simulink model "c8t6_antipark_svpwm"  (R2018b)
settings: Solver=FixedStepDiscrete  StartTime=0.0  StopTime=2  FixedStep=0.000001  RelTol=1e-3
libraries: simulink x1
settings Model: Creator=ganlu  LastModifiedBy=ganlu

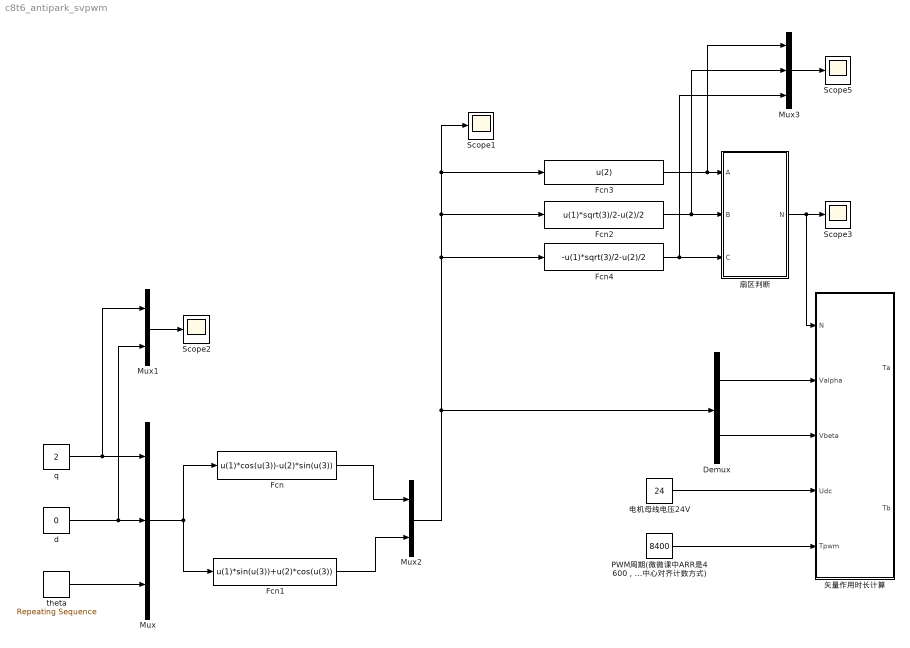
== system c8t6_antipark_svpwm ==
  Demux : Demux  Outputs=2
  Fcn : Fcn  Expr=u(1)*cos(u(3))-u(2)*sin(u(3))
  Fcn1 : Fcn  Expr=u(1)*sin(u(3))+u(2)*cos(u(3))
  Fcn2 : Fcn  Expr=u(1)*sqrt(3)/2-u(2)/2
  Fcn3 : Fcn  Expr=u(2)
  Fcn4 : Fcn  Expr=-u(1)*sqrt(3)/2-u(2)/2
  Mux : Mux  Inputs=3
  Mux1 : Mux  Inputs=2
  Mux2 : Mux  Inputs=2
  Mux3 : Mux  Inputs=3
  "PWM周期(微微课中ARR是4600，中心对齐计数方式) " : Constant  Value=8400
  Scope{1..3,5} (4 alike) : Scope
  d : Constant  Value=0
  q : Constant  Value=2
  theta : simulink/Sources/Repeating Sequence  rep_seq_t=[0 1]  rep_seq_y=[0 2*pi]
  扇区判断 : MATLAB Function  TreatAsAtomicUnit=on
  电机母线电压24V : Constant  Value=24
  矢量作用时长计算 : MATLAB Function  TreatAsAtomicUnit=on
  wires:
  q/1 -> Mux1/1, Mux/1
  d/1 -> Mux1/2, Mux/2
  theta/1 -> Mux/3
  Mux/1 -> Fcn1/1, Fcn/1
  Mux1/1 -> Scope2/1
  Fcn1/1 -> Mux2/2
  Mux2/1 -> Fcn3/1, Scope1/1, Fcn2/1, Fcn4/1, Demux/1
  Fcn/1 -> Mux2/1
  Fcn3/1 -> Mux3/1, 扇区判断/1(A)
  扇区判断/1(N) -> 矢量作用时长计算/1(N), Scope3/1
  Fcn4/1 -> Mux3/3, 扇区判断/3(C)
  Fcn2/1 -> Mux3/2, 扇区判断/2(B)
  Mux3/1 -> Scope5/1
  Demux/1 -> 矢量作用时长计算/2(Valpha)
  Demux/2 -> 矢量作用时长计算/3(Vbeta)
  电机母线电压24V/1 -> 矢量作用时长计算/4(Udc)
  "PWM周期(微微课中ARR是4600，中心对齐计数方式) "/1 -> 矢量作用时长计算/5(Tpwm)

== matlab function c8t6_antipark_svpwm/矢量作用时长计算 ==
  data: N input; Ta output; Valpha input; Vbeta input; Udc input; Tpwm input; Tb output
function [Ta , Tb] = VecatorCalculate(N, Valpha, Vbeta, Udc, Tpwm)

== matlab function c8t6_antipark_svpwm/扇区判断 ==
  data: A input; N output; B input; C input
function N = SectorJudge(A,B,C)

 
N =0;
if(A > 0)
    N = N + 1;
end
if(B > 0)
    N = N + 2;
end
if(C > 0)
    N = N + 4;
end
